simulink model "closed_circuited_cooling_tower_V2011"  (Simulink 7.0)
settings: Solver=ode45  StartTime=3600*24*250  StopTime=3600*24*260  RelTol=1e-3
libraries: carnot x8
settings Model: Creator=Mario  LastModifiedBy=Sandra  SimulationMode=accelerator

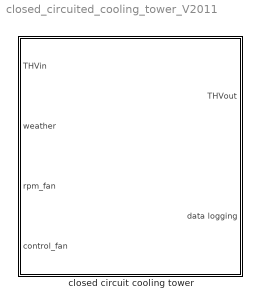
== system closed_circuited_cooling_tower_V2011 ==
  closed circuit cooling tower : Subsystem  AncestorBlock=carnot/misc/THV_template
      mask Type: Closed Circuit Cooling Tower
      mask Description:
      | performance data
      | wet-bulb temperature - 15°C ... 24°C
      | rpm fan - 248 1/min (30%) ... 824 1/min (100%)
      | fluid temperature - 26°C ... 44°C
      | fluid flow rate - 1,07 l/s ... 3,03 l/s
      | water/glykol - 0 % ... 100%
      | 
      | data logging:
      | wet-bulb temperature....[°C]   (ambient air)
      | rpm fan.........................[%]
      | v_dot fan......................[m³/s]
      | rpm fan.........................[1/min]
      | rel_hum.........................[%]     (ambient air)
      | t_air..............................[°C]    (ambient air)
      | energy ct......................[kJ]    (fan motor + recirculating spray pump)
      | power ct.......................[kW]    (fan motor + recirculating spray pump)
      | water consumption.......[kg]
      | Tnodes.........................[°C]    (inactivity modul)
      | THVout
      mask Display:
      | plot(-20,5,140,80,[20 90 90 20 20],[20 20 70 70 20])
      | plot([30 35],[62 65],[40 35],[62 65],[35 35],[62 65],[80 80],[62 65],[75 80],[62 65],[85 80],[62 65],[57 57],[62 65],[52 57],[62 65],[62 57],[62 65])
      | plot([15 20],[22 22],[15 80],[65 65],[15 15],[22 65],[20 90],[24 24])
      | plot([25 100],[58 58],[25 100],[44 44],[60 25],[51 58],[60 25],[51 44])
      | plot([87 93],[36 36],[87 93],[28 28],[87 82],[36 34],[93 98],[36 34],[87 82],[28 30],[93 98],[28 30],[82 82],[34 30],[98 98],[34 30],[82 95],[34 35],[82 95],[30 29])
      | plot([86 90],[32 32],[90 93],[32 33.5],[90 93],[32 30.5])

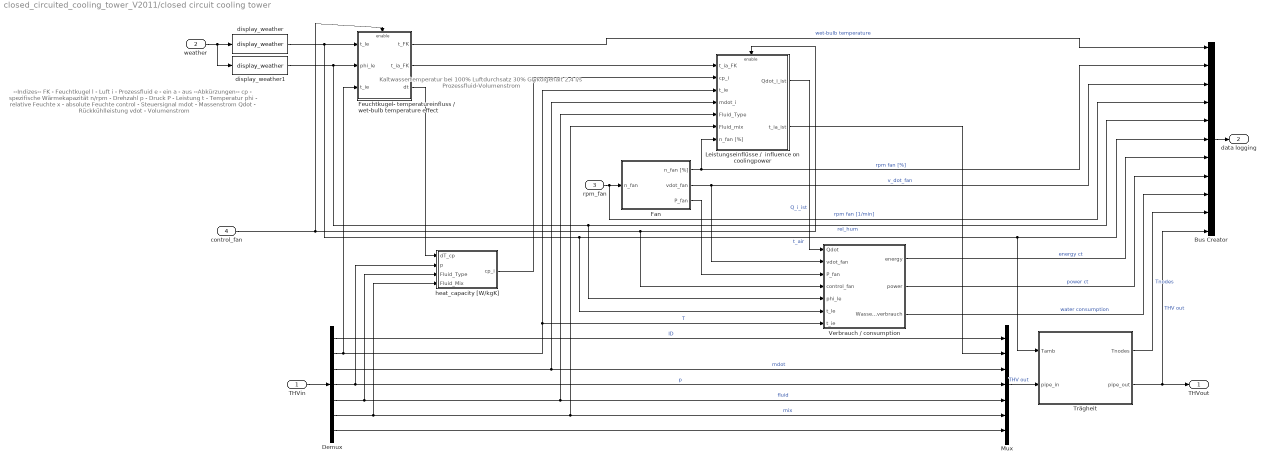
== system closed_circuited_cooling_tower_V2011/closed circuit cooling tower ==
  note: Kaltwassertemperatur bei
      | 100% Luftdurchsatz
      | 30% Glykolgehalt
      | 2,4 l/s Prozessfluid-Volumenstrom
  note: --Indizes--
      | FK - Feuchtkugel
      | l - Luft
      | i - Prozessfluid
      | e - ein
      | a - aus
      |
      |
      | --Abkürzungen--
      | cp - spezifische Wärmekapazität
      | n/rpm - Drehzahl
      | p - Druck
      | P - Leistung
      | t - Temperatur
      | phi - relative Feuchte
      | x - absolute Feuchte
      | control - Steuersignal
      | mdot - Massenstrom
      | Qdot - Rückkühlleistung
      | vdot - Volumenstrom
  THVin : Inport  OutDataType=sfix(16)  OutScaling=2^0
  weather : Inport  Port=2  OutDataType=sfix(16)  OutScaling=2^0
  rpm_fan : Inport  Port=3  OutDataType=sfix(16)  OutScaling=2^0
  control_fan : Inport  Port=4  OutDataType=sfix(16)  OutScaling=2^0
  Bus Creator : BusCreator  Inputs=11
  Demux : Demux  Outputs=[1 1 1 1 1 1 14]
  Fan : Subsystem  AncestorBlock=carnot/misc/THV_template
  Feuchtkugel- temperatureinfluss / wet-bulb temperature effect : Subsystem  AncestorBlock=carnot/misc/THV_template
  Leistungseinflüsse /  influence on coolingpower : Subsystem  AncestorBlock=carnot/misc/THV_template
  Mux : Mux  Inputs=7
  Trägheit : Subsystem  AncestorBlock=carnot/storage/storage_multiport_2  mask(storage with heat exchangers){diameter=0.1, vol=0.04, pos=standing cylinder, heatloss=7, hlossbot=7, axialcond=1.1, tinitial=21}
      mask prompts: diameter "diameter [m]"; vol "volume [m³]"; pos "position"; heatloss "heat loss coefficient wall [W/(m²*K)]"; hlossbot "heat loss coefficient bottom [W/(m²*K)]"; axialcond "effective axial conductivity in [W/(m*K)]"; tinitial "initial temperature [degree centigrade]"
      mask help:
      | Storage is a standing cylinder. It can be divided in several nodes.
      | Outputs can be refined up to nodes temperature sensors.
      | (See mask of storage in subsystem by <look under mask - command> for details of numerical properties).
      |
      | Axial conductivity includes the fluid and wall conductivity.
      | Heat losses are calculated also for top and bottom surfaces.
      mask Help: eval('man(''storage_multiport'')')
      mask StyleString: edit,edit,popup(lying cylinder|standing cylinder),edit,edit,edit,edit
      mask Display: plot(0,0,100,100,[36,36,40,50,54,54,50,40,36],[90,50,45,45,50,90,93,93,90],[36,51,40,51,36],[74,74,79,85,85],[36,51,44,51,36],[54,54,56,58,58])
  Verbrauch / consumption : Subsystem  AncestorBlock=carnot/misc/THV_template
  display_weather : carnot/outputs/display_weather  SystemSampleTime=-1  pos=off  rad=off  ta=on  ts=off  pre=off  rh=off  ci=off  p=off  ws=off  wd=off  col=off
  display_weather1 : carnot/outputs/display_weather  SystemSampleTime=-1  pos=off  rad=off  ta=off  ts=off  pre=off  rh=on  ci=off  p=off  ws=off  wd=off  col=off
  heat_capacity [W/kgK] : Subsystem  AncestorBlock=carnot/materials/heat_capacity
      mask Type: heat capacity
      mask Description:
      | Calculates the  heat_capacity of fluids [J/(kg*K)].
      | Calls calls the function "hcap" in the CARNOT library "carlib".
      | Definition of the fluid types
      | fluid-ID  material           remarks on fluid mix
      | 1           water              vapourcontent in the 2-phase region
      | 2           air                   is (kg water) / (kg air)
      | 3           cotton oil
      | 4           silicone oil
      | 5           water-glycol    gives the volume partition [0..1] of glycol
      mask Help: eval('htmlhelp (''chap_4_2h.htm#heat_capacity'')')
  THVout : Outport  OutDataType=sfix(16)  OutScaling=2^0  InitialOutput=0
  data logging : Outport  Port=2  OutDataType=sfix(16)  OutScaling=2^0  InitialOutput=0
  wires:
  THVin/1 -> Demux/1
  Demux/3 -> Leistungseinflüsse /  influence on coolingpower/4(mdot_i), Mux/3  "mdot"
  Demux/7 -> Mux/7
  Demux/5 -> heat_capacity [W/kgK]/3(Fluid_Type), Mux/5, Leistungseinflüsse /  influence on coolingpower/5(Fluid_Type)  "fluid"
  Mux/1 -> Trägheit/2(pipe_in)  "THV out"
  Demux/4 -> heat_capacity [W/kgK]/2(p), Mux/4  "p"
  rpm_fan/1 -> Fan/1(n_fan), Bus Creator/4  "rpm fan [1/min]"
  Feuchtkugel- temperatureinfluss / wet-bulb temperature effect/3(dt) -> heat_capacity [W/kgK]/1(dT_cp)
  Feuchtkugel- temperatureinfluss / wet-bulb temperature effect/2(t_ia_FK) -> Leistungseinflüsse /  influence on coolingpower/1(t_ia_FK)
  Demux/2 -> Feuchtkugel- temperatureinfluss / wet-bulb temperature effect/3(t_ie), Leistungseinflüsse /  influence on coolingpower/3(t_ie), Verbrauch / consumption/7(t_ie)  "T"
  Leistungseinflüsse /  influence on coolingpower/2(t_ia_ist) -> Mux/2
  heat_capacity [W/kgK]/1(cp_i) -> Leistungseinflüsse /  influence on coolingpower/2(cp_i)
  Fan/2(vdot_fan) -> Verbrauch / consumption/2(vdot_fan), Bus Creator/3  "v_dot_fan"
  Verbrauch / consumption/2(power) -> Bus Creator/8  "power ct"
  Fan/3(P_fan) -> Verbrauch / consumption/3(P_fan)
  control_fan/1 -> Verbrauch / consumption/4(control_fan), Leistungseinflüsse /  influence on coolingpower/Enable, Feuchtkugel- temperatureinfluss / wet-bulb temperature effect/Enable
  Demux/1 -> Mux/1  "ID"
  Feuchtkugel- temperatureinfluss / wet-bulb temperature effect/1(t_FK) -> Bus Creator/1  "wet-bulb temperature"
  Leistungseinflüsse /  influence on coolingpower/1(Qdot_i_ist) -> Verbrauch / consumption/1(Qdot)  "Q_i_ist"
  Fan/1(n_fan [%]) -> Leistungseinflüsse /  influence on coolingpower/7(n_fan [%]), Bus Creator/2  "rpm fan [%]"
  display_weather1/1 -> Feuchtkugel- temperatureinfluss / wet-bulb temperature effect/2(phi_le), Verbrauch / consumption/5(phi_le), Bus Creator/5  "rel_hum"
  display_weather/1 -> Feuchtkugel- temperatureinfluss / wet-bulb temperature effect/1(t_le), Verbrauch / consumption/6(t_le), Trägheit/1(Tamb), Bus Creator/6  "t_air"
  Verbrauch / consumption/3(Wasserverbrauch) -> Bus Creator/9  "water consumption"
  Trägheit/1(Tnodes) -> Bus Creator/10  "Tnodes"
  Trägheit/2(pipe_out) -> THVout/1, Bus Creator/11  "THV out"
  Demux/6 -> heat_capacity [W/kgK]/4(Fluid_Mix), Leistungseinflüsse /  influence on coolingpower/6(Fluid_mix), Mux/6  "mix"
  weather/1 -> display_weather/1, display_weather1/1
  Bus Creator/1 -> data logging/1
  Verbrauch / consumption/1(energy) -> Bus Creator/7  "energy ct"

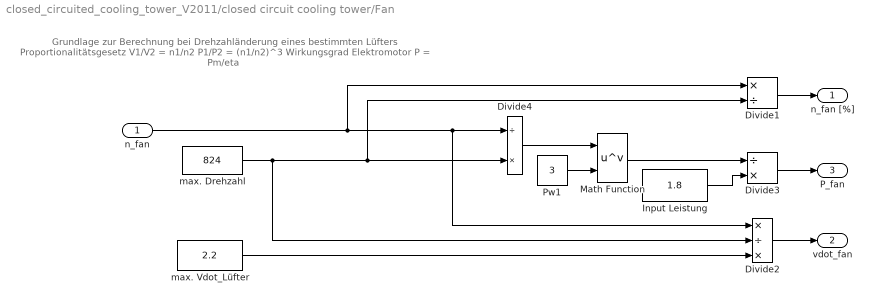
== system closed_circuited_cooling_tower_V2011/closed circuit cooling tower/Fan ==
  note: Grundlage zur Berechnung
      | bei Drehzahländerung eines bestimmten Lüfters
      |
      | Proportionalitätsgesetz
      | V1/V2 = n1/n2
      | P1/P2 = (n1/n2)^3
      |
      | Wirkungsgrad Elektromotor
      | P = Pm/eta
  n_fan : Inport  OutDataType=sfix(16)  OutScaling=2^0
  Divide1 : Product  Inputs=*/  OutDataType=sfix(16)  OutScaling=2^-10
  Divide2 : Product  Inputs=*/*  OutDataType=sfix(16)  OutScaling=2^-10
  Divide3 : Product  Inputs=/*  OutDataType=sfix(16)  OutScaling=2^-10
  Divide4 : Product  Inputs=/*  OutDataType=sfix(16)  OutScaling=2^-10
  Input Leistung : Constant  Value=1.8  OutDataType=sfix(16)  OutScaling=2^0
  Math Function : Math  Operator=pow  OutDataType=sfix(16)  OutScaling=2^0  SaturateOnIntegerOverflow=on
  Pw1 : Constant  Value=3  OutDataType=sfix(16)  OutScaling=2^0
  max. Drehzahl : Constant  Value=824  OutDataType=sfix(16)  OutScaling=2^0
  max. Vdot_Lüfter : Constant  Value=2.2  OutDataType=sfix(16)  OutScaling=2^0
  n_fan [%] : Outport  OutDataType=sfix(16)  OutScaling=2^0  InitialOutput=0
  vdot_fan : Outport  Port=2  OutDataType=sfix(16)  OutScaling=2^0  InitialOutput=0
  P_fan : Outport  Port=3  OutDataType=sfix(16)  OutScaling=2^0  InitialOutput=0
  wires:
  n_fan/1 -> Divide2/1, Divide4/1, Divide1/1
  max. Drehzahl/1 -> Divide2/2, Divide1/2, Divide4/2
  Divide1/1 -> n_fan [%]/1
  Input Leistung/1 -> Divide3/2
  max. Vdot_Lüfter/1 -> Divide2/3
  Divide2/1 -> vdot_fan/1
  Divide3/1 -> P_fan/1
  Divide4/1 -> Math Function/1
  Math Function/1 -> Divide3/1
  Pw1/1 -> Math Function/2

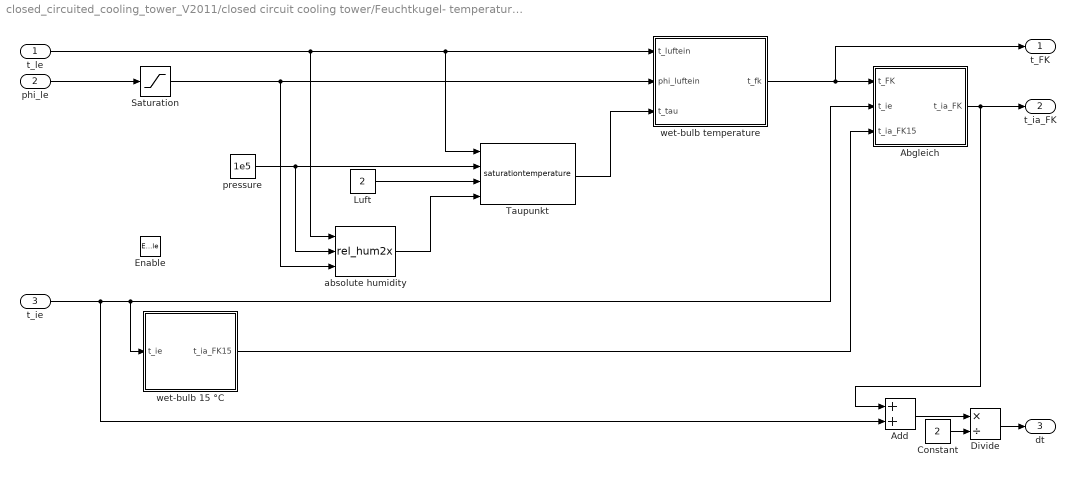
== system closed_circuited_cooling_tower_V2011/closed circuit cooling tower/Feuchtkugel- temperatureinfluss / wet-bulb temperature effect ==
  t_le : Inport  OutDataType=sfix(16)  OutScaling=2^0
  phi_le : Inport  Port=2  OutDataType=sfix(16)  OutScaling=2^0
  t_ie : Inport  Port=3  OutDataType=sfix(16)  OutScaling=2^0
  Enable : EnablePort
  "Abgleich " : Subsystem  AncestorBlock=carnot/misc/THV_template
  Add : Sum  OutDataType=sfix(16)  OutScaling=2^-10
  Constant : Constant  Value=2  OutDataType=sfix(16)  OutScaling=2^0
  Divide : Product  Inputs=*/  OutDataType=sfix(16)  OutScaling=2^-10
  Luft : Constant  Value=2  OutDataType=sfix(16)  OutScaling=2^0
  Saturation : Saturate  UpperLimit=99.0  LowerLimit=0  OutDataType=sfix(16)  OutScaling=2^0
  Taupunkt : carnot/materials/saturationtemperature  SystemSampleTime=-1
  absolute humidity : carnot/basics/rel_hum2x  SystemSampleTime=-1
  pressure : Constant  Value=1e5  OutDataType=sfix(16)  OutScaling=2^0
  wet-bulb 15 °C : Subsystem  AncestorBlock=carnot/misc/THV_template
  wet-bulb temperature : Stateflow chart
  t_FK : Outport  OutDataType=sfix(16)  OutScaling=2^0  InitialOutput=0
  t_ia_FK : Outport  Port=2  OutDataType=sfix(16)  OutScaling=2^0  InitialOutput=0
  dt : Outport  Port=3  OutDataType=sfix(16)  OutScaling=2^0  InitialOutput=0
  wires:
  wet-bulb 15 °C/1(t_ia_FK15) -> "Abgleich "/3(t_ia_FK15)
  wet-bulb temperature/1(t_fk) -> "Abgleich "/1(t_FK), t_FK/1
  t_ie/1 -> Add/2, wet-bulb 15 °C/1(t_ie), "Abgleich "/2(t_ie)
  phi_le/1 -> Saturation/1
  t_le/1 -> Taupunkt/1, wet-bulb temperature/1(t_luftein), absolute humidity/1
  "Abgleich "/1(t_ia_FK) -> Add/1, t_ia_FK/1
  Add/1 -> Divide/1
  Constant/1 -> Divide/2
  Divide/1 -> dt/1
  Saturation/1 -> absolute humidity/3, wet-bulb temperature/2(phi_luftein)
  absolute humidity/1 -> Taupunkt/4
  Luft/1 -> Taupunkt/3
  pressure/1 -> Taupunkt/2, absolute humidity/2
  Taupunkt/1 -> wet-bulb temperature/3(t_tau)

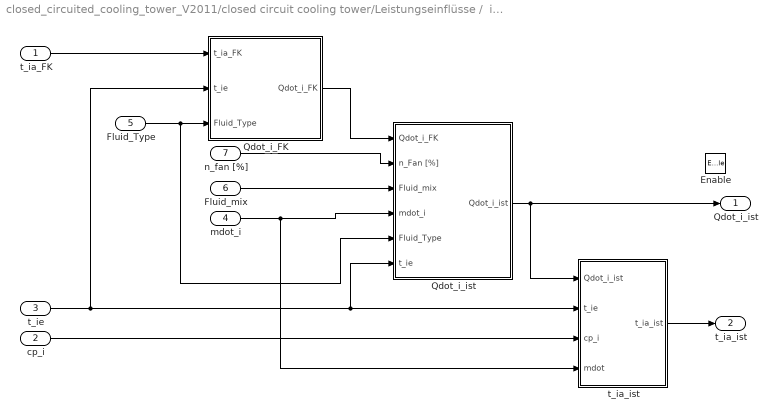
== system closed_circuited_cooling_tower_V2011/closed circuit cooling tower/Leistungseinflüsse /  influence on coolingpower ==
  t_ia_FK : Inport  OutDataType=sfix(16)  OutScaling=2^0
  cp_i : Inport  Port=2  OutDataType=sfix(16)  OutScaling=2^0
  t_ie : Inport  Port=3  OutDataType=sfix(16)  OutScaling=2^0
  mdot_i : Inport  Port=4  OutDataType=sfix(16)  OutScaling=2^0
  Fluid_Type : Inport  Port=5  OutDataType=sfix(16)  OutScaling=2^0
  Fluid_mix : Inport  Port=6  OutDataType=sfix(16)  OutScaling=2^0
  n_fan [%] : Inport  Port=7  OutDataType=sfix(16)  OutScaling=2^0
  Enable : EnablePort
  Qdot_i_FK : Subsystem  AncestorBlock=carnot/misc/THV_template
  "Qdot_i_ist " : Subsystem  AncestorBlock=carnot/misc/THV_template
  "t_ia_ist " : Subsystem  AncestorBlock=carnot/misc/THV_template
  Qdot_i_ist : Outport  OutDataType=sfix(16)  OutScaling=2^0  InitialOutput=0
  t_ia_ist : Outport  Port=2  OutDataType=sfix(16)  OutScaling=2^0  InitialOutput=0
  wires:
  "Qdot_i_ist "/1(Qdot_i_ist) -> Qdot_i_ist/1, "t_ia_ist "/1(Qdot_i_ist)
  Qdot_i_FK/1(Qdot_i_FK) -> "Qdot_i_ist "/1(Qdot_i_FK)
  t_ie/1 -> Qdot_i_FK/2(t_ie), "t_ia_ist "/2(t_ie), "Qdot_i_ist "/6(t_ie)
  t_ia_FK/1 -> Qdot_i_FK/1(t_ia_FK)
  n_fan [%]/1 -> "Qdot_i_ist "/2(n_Fan [%])
  "t_ia_ist "/1(t_ia_ist) -> t_ia_ist/1
  cp_i/1 -> "t_ia_ist "/3(cp_i)
  Fluid_Type/1 -> Qdot_i_FK/3(Fluid_Type), "Qdot_i_ist "/5(Fluid_Type)
  mdot_i/1 -> "Qdot_i_ist "/4(mdot_i), "t_ia_ist "/4(mdot)
  Fluid_mix/1 -> "Qdot_i_ist "/3(Fluid_mix)

== system closed_circuited_cooling_tower_V2011/closed circuit cooling tower/Trägheit ==
  Tamb : Inport  OutDataType=sfix(16)  OutScaling=2^0
  pipe_in : Inport  Port=2  OutDataType=sfix(16)  OutScaling=2^0
  Terminator : Terminator
  multiport storage : Subsystem  mask(internal mask of storage for numerical values){nodes=10, sensors=10, nport=1, d=[diameter vol], u=[heatloss hlossbot], axialcond=axialcond, tinitial=tinitial, pos=pos}
      mask prompts: nodes "number of nodes"; sensors "number of temperature sensors (first is at bottom)"; nport "number of ports"; d "geometry (DO NOT CHANGE HERE)"; u "heat losses (DO NOT CHANGE HERE)"; axialcond "effecive axial conductivity W/(m*K) (DO NOT CHANGE HERE)"; tinitial "initial temperature in °C (DO NOT CHANGE HERE)"; pos "position (DO NOT CHANGE HERE)"
      mask help: Model is one dimesional with <nodes> horizontal slices. Output sensor-temperatures are in equal distances over the storage (first output is lowest node).
      mask init:
      | nodes = max(nodes, 1);
      | sensors = max(sensors, 1);
      | d(1) = max(d(1), 0.001);
      | d(2) = max(d(2), 0.001);
      | pos = pos-1;
      mask Help:
      | The flow is calculated by the upwind scheme heat conduction between nodes by central diffenences (Patankar 1980).
      | Heat exchanger does not have any capacity for the fluid. Heat transfer to storage is calculated per stroage node by an energy balance. Heat transfer coefficient for heat exchanger is calculated from Nu = 0.5*(Gr*Pr)^0.25.
      | Can be charged and discharged by ports (straight incomming pipe, heat exchanger). For the moment You have to add the inports and outports yourself in  the subsystem when changing the number of ports. Be sure to keep the size of the demux after the s-funtion as [sensors 2  2  2] (repeat 2 as many ports as You have).
      mask StyleString: edit,edit,popup(1|2|3|4|5|6|7|8|9|10),edit,edit,edit,edit,edit
  pipe connection to store1 : Subsystem  AncestorBlock=carnot/storage/ports for your storage construction/pipe connection to store  mask(pipe connection to storage){hin=0, hout=1}
      mask prompts: hin "relative height of inlet"; hout "relative height of outlet"
      mask help:
      | The block transforms the incoming THV vector to a vector which the storage interprets as a flow into the storage fluid.
      | Give inlet- and outlet-height as a relative position from 0 (= bottom) to 1 (= top).
      mask init:
      | hin = min(1, max(0, hin));
      | hout = min(1, max(0, hout));
      mask Help: eval('man(''pipe_connection_to_store'')')
  Tnodes : Outport  OutDataType=sfix(16)  OutScaling=2^0  InitialOutput=0
  pipe_out : Outport  Port=2  OutDataType=sfix(16)  OutScaling=2^0  InitialOutput=0
  wires:
  multiport storage/2(Energy) -> Terminator/1
  pipe_in/1 -> pipe connection to store1/2(THVin)
  pipe connection to store1/2(THVout) -> pipe_out/1
  Tamb/1 -> multiport storage/1(Tamb)
  multiport storage/1(Tnodes) -> Tnodes/1
  multiport storage/3("[T p]1") -> pipe connection to store1/1(from store)
  pipe connection to store1/1(to store) -> multiport storage/2(port1)

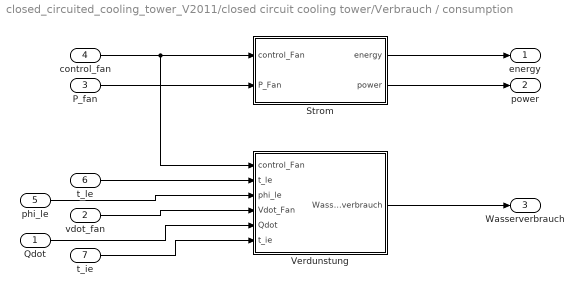
== system closed_circuited_cooling_tower_V2011/closed circuit cooling tower/Verbrauch / consumption ==
  Qdot : Inport  OutDataType=sfix(16)  OutScaling=2^0
  vdot_fan : Inport  Port=2  OutDataType=sfix(16)  OutScaling=2^0
  P_fan : Inport  Port=3  OutDataType=sfix(16)  OutScaling=2^0
  control_fan : Inport  Port=4  OutDataType=sfix(16)  OutScaling=2^0
  phi_le : Inport  Port=5  OutDataType=sfix(16)  OutScaling=2^0
  t_le : Inport  Port=6  OutDataType=sfix(16)  OutScaling=2^0
  t_ie : Inport  Port=7  OutDataType=sfix(16)  OutScaling=2^0
  Strom : Subsystem  AncestorBlock=carnot/misc/THV_template
  Verdunstung : Subsystem  AncestorBlock=carnot/misc/THV_template
  energy : Outport  OutDataType=sfix(16)  OutScaling=2^0  InitialOutput=0
  power : Outport  Port=2  OutDataType=sfix(16)  OutScaling=2^0  InitialOutput=0
  Wasserverbrauch : Outport  Port=3  OutDataType=sfix(16)  OutScaling=2^0  InitialOutput=0
  wires:
  control_fan/1 -> Strom/1(control_Fan), Verdunstung/1(control_Fan)
  P_fan/1 -> Strom/2(P_Fan)
  Strom/2(power) -> power/1
  t_le/1 -> Verdunstung/2(t_le)
  Verdunstung/1(Wasserverbrauch) -> Wasserverbrauch/1
  phi_le/1 -> Verdunstung/3(phi_le)
  vdot_fan/1 -> Verdunstung/4(Vdot_Fan)
  Qdot/1 -> Verdunstung/5(Qdot)
  t_ie/1 -> Verdunstung/6(t_ie)
  Strom/1(energy) -> energy/1

== system closed_circuited_cooling_tower_V2011/closed circuit cooling tower/heat_capacity [W/kgK] ==
  dT_cp : Inport  OutDataType=sfix(16)  OutScaling=2^0
  p : Inport  Port=2  OutDataType=sfix(16)  OutScaling=2^0
  Fluid_Type : Inport  Port=3  OutDataType=sfix(16)  OutScaling=2^0
  Fluid_Mix : Inport  Port=4  OutDataType=sfix(16)  OutScaling=2^0
  S-Function : S-Function  FunctionName=capfluid
  cp_i : Outport  OutDataType=sfix(16)  OutScaling=2^0  InitialOutput=0
  wires:
  S-Function/1 -> cp_i/1
  Fluid_Type/1 -> S-Function/1
  Fluid_Mix/1 -> S-Function/2
  dT_cp/1 -> S-Function/3
  p/1 -> S-Function/4

== system closed_circuited_cooling_tower_V2011/closed circuit cooling tower/Feuchtkugel- temperatureinfluss / wet-bulb temperature effect/Abgleich  ==
  note: Durch den Abgleich der vorliegenden Datensätze
      | wierd die Annahme getroffen
      | das bei einer reduzierung der Feuchtkugeltemp um 1K
      |  sich die Kaltwassertemp um 0.27K sinkt.
      |
      | y = ((t_FK-15)*0.27)+t_ia_100
      |
      | Ab eine Eintritstemperatur von 41 °C wierd mit
      | dem Faktor 0,25 K gerechnet.
      |
      | y = ((t_FK-15)*0.25)+t_ia_100
  t_FK : Inport  OutDataType=sfix(16)  OutScaling=2^0
  t_ie : Inport  Port=2  OutDataType=sfix(16)  OutScaling=2^0
  t_ia_FK15 : Inport  Port=3  OutDataType=sfix(16)  OutScaling=2^0
  Embedded MATLAB Function : Stateflow chart
  t_ia_FK : Outport  OutDataType=sfix(16)  OutScaling=2^0  InitialOutput=0
  wires:
  Embedded MATLAB Function/1(y) -> t_ia_FK/1
  t_FK/1 -> Embedded MATLAB Function/1(t_fk)
  t_ia_FK15/1 -> Embedded MATLAB Function/2(t_ia_fk15)
  t_ie/1 -> Embedded MATLAB Function/3(t_ie)

== system closed_circuited_cooling_tower_V2011/closed circuit cooling tower/Feuchtkugel- temperatureinfluss / wet-bulb temperature effect/wet-bulb 15 °C ==
  t_ie : Inport  OutDataType=sfix(16)  OutScaling=2^0
  Lookup Table : Lookup  InputValues=[26 28 30 32 34 36 38 40 42 44 79.2]  Table=[22.6 23.9 25.2 26.4 27.7 28.9 30.1 31.2 32.4 33.5 49.25]  OutDataType=sfix(16)  OutScaling=2^0
  t_ia_FK15 : Outport  OutDataType=sfix(16)  OutScaling=2^0  InitialOutput=0
  wires:
  t_ie/1 -> Lookup Table/1
  Lookup Table/1 -> t_ia_FK15/1

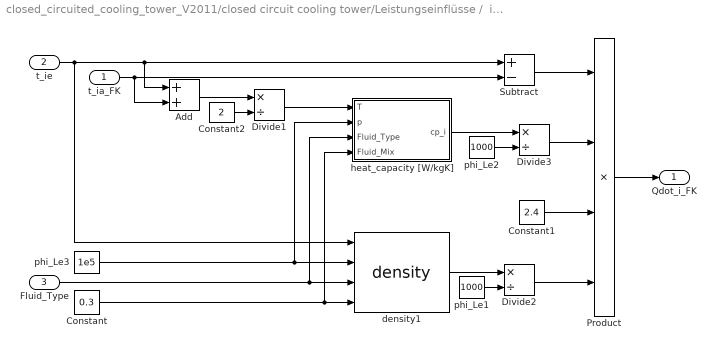
== system closed_circuited_cooling_tower_V2011/closed circuit cooling tower/Leistungseinflüsse /  influence on coolingpower/Qdot_i_FK ==
  t_ia_FK : Inport  OutDataType=sfix(16)  OutScaling=2^0
  t_ie : Inport  Port=2  OutDataType=sfix(16)  OutScaling=2^0
  Fluid_Type : Inport  Port=3  OutDataType=sfix(16)  OutScaling=2^0
  Add : Sum  OutDataType=sfix(16)  OutScaling=2^-10
  Constant : Constant  Value=0.3  OutDataType=sfix(16)  OutScaling=2^0
  Constant1 : Constant  Value=2.4  OutDataType=sfix(16)  OutScaling=2^0
  Constant2 : Constant  Value=2  OutDataType=sfix(16)  OutScaling=2^0
  Divide1 : Product  Inputs=*/  OutDataType=sfix(16)  OutScaling=2^-10
  Divide2 : Product  Inputs=*/  OutDataType=sfix(16)  OutScaling=2^-10
  Divide3 : Product  Inputs=*/  OutDataType=sfix(16)  OutScaling=2^-10
  Product : Product  Inputs=4  OutDataType=sfix(16)  OutScaling=2^0  RndMeth=Zero
  Subtract : Sum  Inputs=+-  OutDataType=sfix(16)  OutScaling=2^-10
  density1 : carnot/materials/density  SystemSampleTime=-1
  heat_capacity [W/kgK] : Subsystem  AncestorBlock=carnot/materials/heat_capacity
      mask Type: heat capacity
      mask Description:
      | Calculates the  heat_capacity of fluids [J/(kg*K)].
      | Calls calls the function "hcap" in the CARNOT library "carlib".
      | Definition of the fluid types
      | fluid-ID  material           remarks on fluid mix
      | 1           water              vapourcontent in the 2-phase region
      | 2           air                   is (kg water) / (kg air)
      | 3           cotton oil
      | 4           silicone oil
      | 5           water-glycol    gives the volume partition [0..1] of glycol
      mask Help: eval('htmlhelp (''chap_4_2h.htm#heat_capacity'')')
  phi_Le1 : Constant  Value=1000  OutDataType=sfix(16)  OutScaling=2^0
  phi_Le2 : Constant  Value=1000  OutDataType=sfix(16)  OutScaling=2^0
  phi_Le3 : Constant  Value=1e5  OutDataType=sfix(16)  OutScaling=2^0
  Qdot_i_FK : Outport  OutDataType=sfix(16)  OutScaling=2^0  InitialOutput=0
  wires:
  t_ia_FK/1 -> Subtract/2, Add/2
  Product/1 -> Qdot_i_FK/1
  Subtract/1 -> Product/1
  t_ie/1 -> density1/1, Subtract/1, Add/1
  Constant/1 -> density1/4, heat_capacity [W/kgK]/4(Fluid_Mix)
  density1/1 -> Divide2/1
  phi_Le3/1 -> density1/2, heat_capacity [W/kgK]/2(p)
  Fluid_Type/1 -> density1/3, heat_capacity [W/kgK]/3(Fluid_Type)
  phi_Le1/1 -> Divide2/2
  Divide2/1 -> Product/4
  Constant1/1 -> Product/3
  heat_capacity [W/kgK]/1(cp_i) -> Divide3/1
  Constant2/1 -> Divide1/2
  Divide1/1 -> heat_capacity [W/kgK]/1(T)
  Add/1 -> Divide1/1
  phi_Le2/1 -> Divide3/2
  Divide3/1 -> Product/2

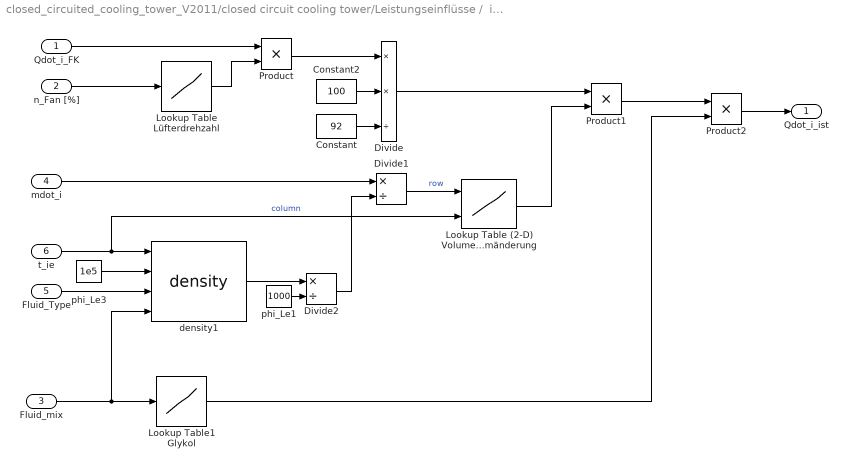
== system closed_circuited_cooling_tower_V2011/closed circuit cooling tower/Leistungseinflüsse /  influence on coolingpower/Qdot_i_ist  ==
  Qdot_i_FK : Inport  OutDataType=sfix(16)  OutScaling=2^0
  n_Fan [%] : Inport  Port=2  OutDataType=sfix(16)  OutScaling=2^0
  Fluid_mix : Inport  Port=3  OutDataType=sfix(16)  OutScaling=2^0
  mdot_i : Inport  Port=4  OutDataType=sfix(16)  OutScaling=2^0
  Fluid_Type : Inport  Port=5  OutDataType=sfix(16)  OutScaling=2^0
  t_ie : Inport  Port=6  OutDataType=sfix(16)  OutScaling=2^0
  Constant : Constant  Value=92  OutDataType=sfix(16)  OutScaling=2^0
  Constant2 : Constant  Value=100  OutDataType=sfix(16)  OutScaling=2^0
  Divide : Product  Inputs=**/  OutDataType=sfix(16)  OutScaling=2^-10
  Divide1 : Product  Inputs=*/  OutDataType=sfix(16)  OutScaling=2^-10
  Divide2 : Product  Inputs=*/  OutDataType=sfix(16)  OutScaling=2^-10
  Lookup Table (2-D) Volumenstromänderung : Lookup2D  RowIndex=[1.07 1.77 2.4 2.65 3.03]  ColumnIndex=[25 30 35 40 45 50 55 60 65]  Table=[0.7248 0.7054 0.6860 0.6666 0.6472 0.6278 0.6084 0.5890 0.5696; 0.9493 0.9294 0.9096 0.8897 0.8698 0.8500 0.8301 0.8103 0.7904; 1 1 1 1 1 1 1 1 1; 1.1191 1.1295 1.0956 1.0674 1.0450 1.0284 1.0175 1.0123 1.0129; 1.2370 1.1910 1.1526 1.1219 1.0988 1.0833 1.0754 1.0752 1.0826]  OutDataType=sfix(16)  OutScaling=2^0
  Lookup Table Lüfterdrehzahl : Lookup  InputValues=[0 0.2 0.3 0.5 0.7 0.9 1]  Table=[0 0.37 0.482 0.625 0.786 0.928 1]  OutDataType=sfix(16)  OutScaling=2^0
  Lookup Table1 Glykol : Lookup  InputValues=[0 0.1 0.2 0.3 0.4 0.5 0.6 0.7 0.8 0.9 1]  Table=[1 0.98 0.95 0.92 0.875 0.83 0.78 0.73 0.68 0.63 0.57]  OutDataType=sfix(16)  OutScaling=2^0
  Product : Product  OutDataType=sfix(16)  OutScaling=2^0  RndMeth=Zero
  Product1 : Product  OutDataType=sfix(16)  OutScaling=2^0  RndMeth=Zero
  Product2 : Product  OutDataType=sfix(16)  OutScaling=2^0  RndMeth=Zero
  density1 : carnot/materials/density  SystemSampleTime=-1
  phi_Le1 : Constant  Value=1000  OutDataType=sfix(16)  OutScaling=2^0
  phi_Le3 : Constant  Value=1e5  OutDataType=sfix(16)  OutScaling=2^0
  Qdot_i_ist : Outport  OutDataType=sfix(16)  OutScaling=2^0  InitialOutput=0
  wires:
  n_Fan [%]/1 -> Lookup Table Lüfterdrehzahl/1
  Lookup Table Lüfterdrehzahl/1 -> Product/2
  Qdot_i_FK/1 -> Product/1
  Product/1 -> Divide/1
  Product1/1 -> Product2/1
  Lookup Table1 Glykol/1 -> Product2/2
  Fluid_mix/1 -> density1/4, Lookup Table1 Glykol/1
  Divide/1 -> Product1/1
  Constant/1 -> Divide/3
  mdot_i/1 -> Divide1/1
  Product2/1 -> Qdot_i_ist/1
  density1/1 -> Divide2/1
  phi_Le3/1 -> density1/2
  Fluid_Type/1 -> density1/3
  phi_Le1/1 -> Divide2/2
  Divide2/1 -> Divide1/2
  t_ie/1 -> density1/1, Lookup Table (2-D) Volumenstromänderung/2  "column"
  Divide1/1 -> Lookup Table (2-D) Volumenstromänderung/1  "row"
  Lookup Table (2-D) Volumenstromänderung/1 -> Product1/2
  Constant2/1 -> Divide/2

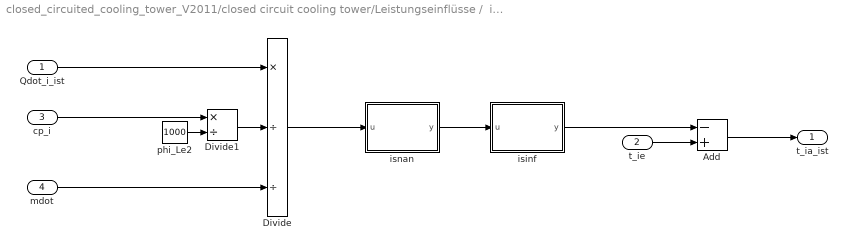
== system closed_circuited_cooling_tower_V2011/closed circuit cooling tower/Leistungseinflüsse /  influence on coolingpower/t_ia_ist  ==
  Qdot_i_ist : Inport  OutDataType=sfix(16)  OutScaling=2^0
  t_ie : Inport  Port=2  OutDataType=sfix(16)  OutScaling=2^0
  cp_i : Inport  Port=3  OutDataType=sfix(16)  OutScaling=2^0
  mdot : Inport  Port=4  OutDataType=sfix(16)  OutScaling=2^0
  Add : Sum  Inputs=-+  OutDataType=sfix(16)  OutScaling=2^-10
  Divide : Product  Inputs=*//  OutDataType=sfix(16)  OutScaling=2^-10
  Divide1 : Product  Inputs=*/  OutDataType=sfix(16)  OutScaling=2^-10
  isinf : Stateflow chart
  isnan : Stateflow chart
  phi_Le2 : Constant  Value=1000  OutDataType=sfix(16)  OutScaling=2^0
  t_ia_ist : Outport  OutDataType=sfix(16)  OutScaling=2^0  InitialOutput=0
  wires:
  Add/1 -> t_ia_ist/1
  Qdot_i_ist/1 -> Divide/1
  t_ie/1 -> Add/2
  Divide/1 -> isnan/1(u)
  cp_i/1 -> Divide1/1
  isnan/1(y) -> isinf/1(u)
  phi_Le2/1 -> Divide1/2
  Divide1/1 -> Divide/2
  mdot/1 -> Divide/3
  isinf/1(y) -> Add/1

== system closed_circuited_cooling_tower_V2011/closed circuit cooling tower/Trägheit/multiport storage ==
  Tamb : Inport  OutDataType=sfix(16)  OutScaling=2^0
  port1 : Inport  Port=2  OutDataType=sfix(16)  OutScaling=2^0
  S-Function : S-Function  FunctionName=store_hx  Parameters="d(1), d(2),  pos, u(1), u(2),  axialcond,  tinitial,  nodes, nport, sensors"
  Tnodes : Outport  OutDataType=sfix(16)  OutScaling=2^0  InitialOutput=0
  Energy : Outport  Port=2  OutDataType=sfix(16)  OutScaling=2^0  InitialOutput=0
  "[T p]1" : Outport  Port=3  OutDataType=sfix(16)  OutScaling=2^0  InitialOutput=0
  wires:
  S-Function/2 -> Energy/1
  S-Function/3 -> "[T p]1"/1
  S-Function/1 -> Tnodes/1
  port1/1 -> S-Function/2
  Tamb/1 -> S-Function/1

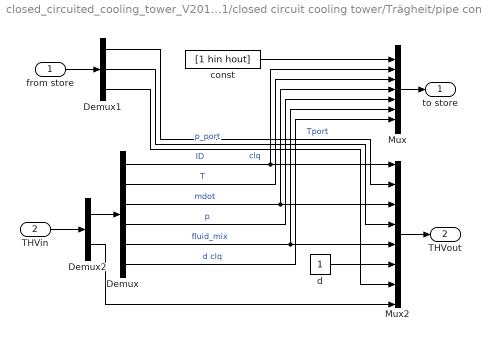
== system closed_circuited_cooling_tower_V2011/closed circuit cooling tower/Trägheit/pipe connection to store1 ==
  from store : Inport  OutDataType=sfix(16)  OutScaling=2^0
  THVin : Inport  Port=2  OutDataType=sfix(16)  OutScaling=2^0
  Demux : Demux  Outputs=[1 1 1 1 2 4]
  Demux1 : Demux  Outputs=[1 1 3]
  Demux2 : Demux  Outputs=[10 -1]
  Mux : Mux  Inputs=7
  Mux2 : Mux  Inputs=8
  const : Constant  Value=[1 hin hout]  OutDataType=sfix(16)  OutScaling=2^0
  d : Constant  OutDataType=sfix(16)  OutScaling=2^0
  to store : Outport  OutDataType=sfix(16)  OutScaling=2^0  InitialOutput=0
  THVout : Outport  Port=2  OutDataType=sfix(16)  OutScaling=2^0  InitialOutput=0
  wires:
  Demux/1 -> Mux/2, Mux2/1  "ID"
  from store/1 -> Demux1/1
  Demux2/1 -> Demux/1
  THVin/1 -> Demux2/1
  Demux/6 -> Mux/7  "d clq"
  Demux/5 -> Mux/6, Mux2/5  "fluid_mix"
  Demux/4 -> Mux/5  "p"
  Demux/3 -> Mux2/3, Mux/4  "mdot"
  Demux/2 -> Mux/3  "T"
  d/1 -> Mux2/6
  const/1 -> Mux/1
  Demux1/2 -> Mux2/4  "p_port"
  Demux1/1 -> Mux2/2  "Tport"
  Demux2/2 -> Mux2/8
  Demux1/3 -> Mux2/7  "clq"
  Mux/1 -> to store/1
  Mux2/1 -> THVout/1

== system closed_circuited_cooling_tower_V2011/closed circuit cooling tower/Verbrauch / consumption/Strom ==
  control_Fan : Inport  OutDataType=sfix(16)  OutScaling=2^0
  P_Fan : Inport  Port=2  OutDataType=sfix(16)  OutScaling=2^0
  Add : Sum  OutDataType=sfix(16)  OutScaling=2^-10
  Integrator1 : Integrator
  Product : Product  OutDataType=sfix(16)  OutScaling=2^0  RndMeth=Zero
  Product2 : Product  Inputs=*/  SaturateOnIntegerOverflow=on  RndMeth=Zero  InputSameDT=on
  Rieselwasserpumpe [kW] : Constant  Value=0.25  OutDataType=sfix(16)  OutScaling=2^0
  factor1 : Constant  Value=3600
  energy : Outport  OutDataType=sfix(16)  OutScaling=2^0  InitialOutput=0
  power : Outport  Port=2  OutDataType=sfix(16)  OutScaling=2^0  InitialOutput=0
  wires:
  Rieselwasserpumpe [kW]/1 -> Add/1
  Product/1 -> power/1, Integrator1/1
  control_Fan/1 -> Product/1
  Add/1 -> Product/2
  P_Fan/1 -> Add/2
  Integrator1/1 -> Product2/1
  factor1/1 -> Product2/2
  Product2/1 -> energy/1

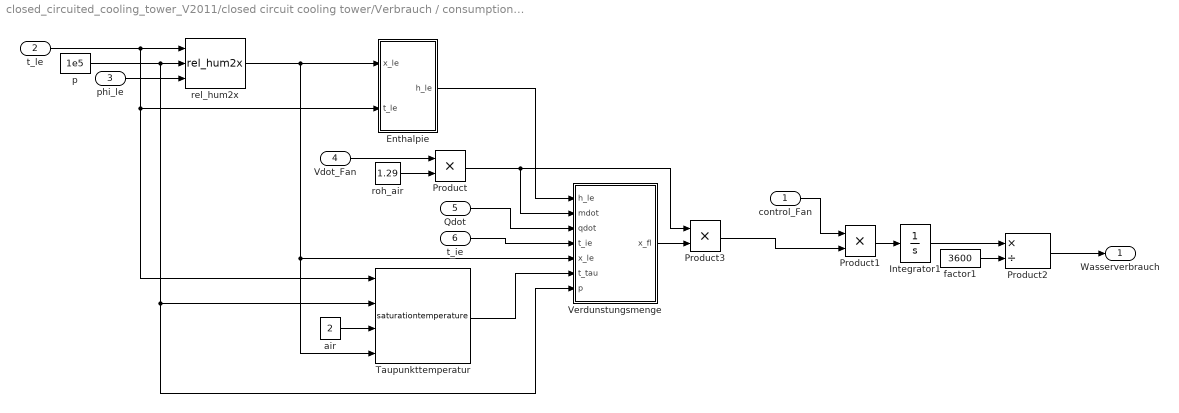
== system closed_circuited_cooling_tower_V2011/closed circuit cooling tower/Verbrauch / consumption/Verdunstung ==
  control_Fan : Inport  OutDataType=sfix(16)  OutScaling=2^0
  t_le : Inport  Port=2  OutDataType=sfix(16)  OutScaling=2^0
  phi_le : Inport  Port=3  OutDataType=sfix(16)  OutScaling=2^0
  Vdot_Fan : Inport  Port=4  OutDataType=sfix(16)  OutScaling=2^0
  Qdot : Inport  Port=5  OutDataType=sfix(16)  OutScaling=2^0
  t_ie : Inport  Port=6  OutDataType=sfix(16)  OutScaling=2^0
  "Enthalpie " : Subsystem  AncestorBlock=carnot/misc/THV_template
  Integrator1 : Integrator
  Product : Product  OutDataType=sfix(16)  OutScaling=2^0  RndMeth=Zero
  Product1 : Product  OutDataType=sfix(16)  OutScaling=2^0  RndMeth=Zero
  Product2 : Product  Inputs=*/  SaturateOnIntegerOverflow=on  RndMeth=Zero  InputSameDT=on
  Product3 : Product  OutDataType=sfix(16)  OutScaling=2^0  RndMeth=Zero
  Taupunkttemperatur : carnot/materials/saturationtemperature  SystemSampleTime=-1
  Verdunstungsmenge : Stateflow chart
  air : Constant  Value=2  OutDataType=sfix(16)  OutScaling=2^0
  factor1 : Constant  Value=3600
  p : Constant  Value=1e5  OutDataType=sfix(16)  OutScaling=2^0
  rel_hum2x : carnot/basics/rel_hum2x  SystemSampleTime=-1
  roh_air : Constant  Value=1.29  OutDataType=sfix(16)  OutScaling=2^0
  Wasserverbrauch : Outport  OutDataType=sfix(16)  OutScaling=2^0  InitialOutput=0
  wires:
  t_le/1 -> rel_hum2x/1, Taupunkttemperatur/1, "Enthalpie "/2(t_le)
  p/1 -> rel_hum2x/2, Taupunkttemperatur/2, Verdunstungsmenge/7(p)
  phi_le/1 -> rel_hum2x/3
  Vdot_Fan/1 -> Product/1
  roh_air/1 -> Product/2
  "Enthalpie "/1(h_le) -> Verdunstungsmenge/1(h_le)
  rel_hum2x/1 -> "Enthalpie "/1(x_le), Taupunkttemperatur/4, Verdunstungsmenge/5(x_le)
  Qdot/1 -> Verdunstungsmenge/3(qdot)
  Taupunkttemperatur/1 -> Verdunstungsmenge/6(t_tau)
  air/1 -> Taupunkttemperatur/3
  Integrator1/1 -> Product2/1
  factor1/1 -> Product2/2
  Product2/1 -> Wasserverbrauch/1
  Product1/1 -> Integrator1/1
  control_Fan/1 -> Product1/1
  Product3/1 -> Product1/2
  Product/1 -> Verdunstungsmenge/2(mdot), Product3/1
  t_ie/1 -> Verdunstungsmenge/4(t_ie)
  Verdunstungsmenge/1(x_fl) -> Product3/2

== system closed_circuited_cooling_tower_V2011/closed circuit cooling tower/Leistungseinflüsse /  influence on coolingpower/Qdot_i_FK/heat_capacity [W/kgK] ==
  T : Inport  OutDataType=sfix(16)  OutScaling=2^0
  p : Inport  Port=2  OutDataType=sfix(16)  OutScaling=2^0
  Fluid_Type : Inport  Port=3  OutDataType=sfix(16)  OutScaling=2^0
  Fluid_Mix : Inport  Port=4  OutDataType=sfix(16)  OutScaling=2^0
  S-Function : S-Function  FunctionName=capfluid
  cp_i : Outport  OutDataType=sfix(16)  OutScaling=2^0  InitialOutput=0
  wires:
  S-Function/1 -> cp_i/1
  Fluid_Type/1 -> S-Function/1
  Fluid_Mix/1 -> S-Function/2
  T/1 -> S-Function/3
  p/1 -> S-Function/4

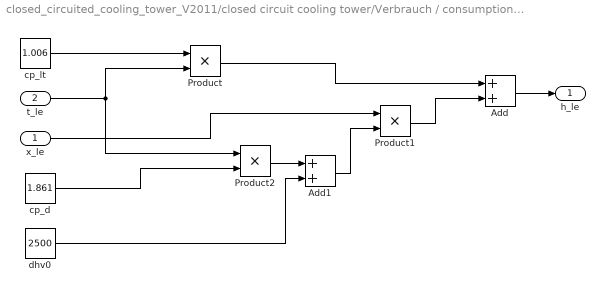
== system closed_circuited_cooling_tower_V2011/closed circuit cooling tower/Verbrauch / consumption/Verdunstung/Enthalpie  ==
  x_le : Inport  OutDataType=sfix(16)  OutScaling=2^0
  t_le : Inport  Port=2  OutDataType=sfix(16)  OutScaling=2^0
  Add : Sum  OutDataType=sfix(16)  OutScaling=2^-10
  Add1 : Sum  OutDataType=sfix(16)  OutScaling=2^-10
  Product : Product  OutDataType=sfix(16)  OutScaling=2^0  RndMeth=Zero
  Product1 : Product  OutDataType=sfix(16)  OutScaling=2^0  RndMeth=Zero
  Product2 : Product  OutDataType=sfix(16)  OutScaling=2^0  RndMeth=Zero
  cp_d : Constant  Value=1.861  OutDataType=sfix(16)  OutScaling=2^0
  cp_lt : Constant  Value=1.006  OutDataType=sfix(16)  OutScaling=2^0
  dhv0 : Constant  Value=2500  OutDataType=sfix(16)  OutScaling=2^0
  h_le : Outport  OutDataType=sfix(16)  OutScaling=2^0  InitialOutput=0
  wires:
  Add/1 -> h_le/1
  cp_lt/1 -> Product/1
  t_le/1 -> Product/2, Product2/1
  Product/1 -> Add/1
  Product1/1 -> Add/2
  x_le/1 -> Product1/1
  cp_d/1 -> Product2/2
  Add1/1 -> Product1/2
  Product2/1 -> Add1/1
  dhv0/1 -> Add1/2

== matlab function closed circuit cooling tower/Feuchtkugel- temperatureinfluss / wet-bulb temperature effect/Abgleich /Embedded MATLAB Function ==
  data: t_fk input inherited; y output inherited; t_ia_fk15 input inherited; t_ie input inherited
%Festlegung der Eingänge
function y = fcn(t_fk, t_ia_fk15, t_ie)

%Änderung des Faktors
if t_ie < 41
    
    y = ((t_fk-15)*0.27)+t_ia_fk15;
    
else
    
    y = ((t_fk-15)*0.25)+t_ia_fk15;
    
end

== matlab function closed circuit cooling tower/Feuchtkugel- temperatureinfluss / wet-bulb temperature effect/wet-bulb temperature ==
  data: t_luftein input inherited; t_fk output inherited; phi_luftein input inherited; t_tau input inherited
%Festlegung der Eingänge
function t_fk = fcn(t_luftein, phi_luftein, t_tau)

%Konstante/Variable
cp_luft = 1.006;        %[kJ/kgK]
cp_dampf = 1.861;       %[kJ/kgK]
cp_wasser = 4.19;       %[kJ/kgK]
dh_v0 = 2500;           %[kJ/kg]
phi_feuchtkugel = 100;  %[%]
p = 10^5;               %[Pa]
m = 1;
tmax = t_luftein;       %[°C]
tmin = t_tau;           %[°C]

% Absolute Feuchte-Berechnung Lufteintritt Bereich 0°C < t < 100°C [1]
ps_luftein = 611*exp((-1.91275)*10^(-4)+7.258*10^(-2)*t_luftein-2.939*10^(-4)*t_luftein^2+9.841*10^(-7)*t_luftein^3-1.92*10^(-9)*t_luftein^4);
x_luftein = (0.622*(phi_luftein/100)*ps_luftein)/(p-(phi_luftein/100)*ps_luftein);

% Enthalpieberechnung Lufteintritt
h_luftein = cp_luft*t_luftein+x_luftein*(cp_dampf*t_luftein+dh_v0);

% Feuchtkugeltemperaturberechnung, Halbierungsverfahren
t_feuchtkugel = (tmax+tmin)/2;

% Absolute Feuchteberechnung Feuchtkugel Bereich 0°C < t < 100°C [1]
ps_feuchtkugel = 611*exp((-1.91275)*10^(-4)+7.258*10^(-2)*t_feuchtkugel-2.939*10^(-4)*t_feuchtkugel^2+9.841*10^(-7)*t_feuchtkugel^3-1.92*10^(-9)*t_feuchtkugel^4);
x_feuchtkugel = (0.622*(phi_feuchtkugel/100)*ps_feuchtkugel)/(p-(phi_feuchtkugel/100)*ps_feuchtkugel);

% Enthalpieberechnung Feuchtkugel
h_feuchtkugel = cp_luft*t_feuchtkugel+x_feuchtkugel*(cp_dampf*t_feuchtkugel+dh_v0);

% Berechnung der Werte u1 und u2,; Formel aus VDI-Wärmeatlas
u1 = (h_luftein-h_feuchtkugel)/(x_luftein-x_feuchtkugel);
u2 = cp_wasser*t_feuchtkugel;

% Bewertung von u1 und u2 Beginn der Schleife
%            (u1-u2)<=0.001 ist die Feuchtkugeltemperatur gefunden
%            u1>u2 tmax = tFk
%            u1<u2 tmin = tFk
 while (u1-u2)>0.001 || (u1-u2)< 0 
    
    if u1>u2
        tmax = t_feuchtkugel;
        
    else 
        tmin = t_feuchtkugel;
        
    end
  
% Feuchtkugeltemperaturberechnung
t_feuchtkugel = (tmax+tmin)/2;

% Absolute Feuchteberechnung Feuchtkugel
ps_feuchtkugel = 611*exp((-1.91275)*10^(-4)+7.258*10^(-2)*t_feuchtkugel-2.939*10^(-4)*t_feuchtkugel^2+9.841*10^(-7)*t_feuchtkugel^3-1.92*10^(-9)*t_feuchtkugel^4);
x_feuchtkugel = (0.622*(phi_feuchtkugel/100)*ps_feuchtkugel)/(p-(phi_feuchtkugel/100)*ps_feuchtkugel);

% Enthalpieberechnung Feuchtkugel
h_feuchtkugel = cp_luft*t_feuchtkugel+x_feuchtkugel*(cp_dampf*t_feuchtkugel+dh_v0);

% Berechnung der Werte u1 und u2
u1 = (h_luftein-h_feuchtkugel)/(x_luftein-x_feuchtkugel);
u2 = cp_wasser*t_feuchtkugel;

% Schleifenzähler
m = m+1;
 
end

% Feuchtkugeltemperatur gefunden - Ausgabe
t_fk = t_feuchtkugel;

== matlab function closed circuit cooling tower/Leistungseinflüsse / influence on coolingpower/t_ia_ist /isinf ==
  data: u input inherited; y output inherited

function y = fcn(u)

%Verhindert die Fehlerausgabe bei Teilen mit dem Wert 0 
%Dieser Zustand tritt ein wenn der Volumenstrom 0 l/s gesetzt wird.

v = isinf (u);

if v == 0
    
    y = u;

else 
    
    y = 0;
    
end

== matlab function closed circuit cooling tower/Leistungseinflüsse / influence on coolingpower/t_ia_ist /isnan ==
  data: u input inherited; y output inherited

function y = fcn(u)

%Verhindert die Fehlerausgabe bei Teilen durch den Wert 0 
%Dieser Zustand tritt ein wenn der Volumenstrom 0 l/s gesetzt wird.

v = isnan (u);

if v == 0
    
    y = u;

else 
    
    y = 0;
    
end

== matlab function closed circuit cooling tower/Verbrauch / consumption/Verdunstung/Verdunstungsmenge ==
  data: h_le input inherited; mdot input inherited; x_fl output inherited; qdot input inherited; t_ie input inherited; x_le input inherited; t_tau input inherited; p input inherited
function x_fl = fcn(h_le, mdot, qdot, t_ie, x_le, t_tau, p)

cp_lt = 1.006;
cp_d = 1.861;
cp_w = 4.19;
dhv0 = 2500;
tmax = t_ie;
tmin = t_tau;
t_zw = 15;
phi_luftaus = 100;
m = 1;


% Vorbedingung qdot muss positiv sein um eine Verdunstung zu gewährleisten ansonsten ist es ein Kondensation
if qdot < 0
    
    x_luftaus = 0;
    
else
    % Luftaustrittstemperaturberechnung, Halbierungsverfahren
        t_luftaus = (tmax+tmin)/2;
    
    % Absolute Feuchte-Berechnung Lufteintritt
        ps_luftaus = 611*exp((-1.91275)*10^(-4)+7.258*10^(-2)*t_luftaus-2.939*10^(-4)*t_luftaus^2+9.841*10^(-7)*t_luftaus^3-1.92*10^(-9)*t_luftaus^4);
        x_luftaus = (0.622*(phi_luftaus/100)*ps_luftaus)/(p-(phi_luftaus/100)*ps_luftaus);

    % Enthalpie Luftaustritt mit dem schon berechneten Qpkt
        h_la = qdot/mdot + (x_luftaus-x_le)*cp_w*t_zw + h_le;
    
    % Austrittstemperatur 
        tlab = (h_la - x_luftaus*dhv0)/(cp_lt + x_luftaus*cp_d);

    % Beginn der Schleife 
    % (t_luftaus - tlab) < 0,001 und > -0,001 ist die Austrittstemperatur gefunden
    %  t_luftaus < tlab  tmin = t_luftaus
    %  t_luftaus > tlab  tmax = t_luftaus
        while (t_luftaus - tlab)>0.001 || (t_luftaus - tlab) < -0.001 && m < 30
    
            if t_luftaus < tlab
        
                tmin = t_luftaus;
    
            else
        
                tmax = t_luftaus;
    
            end
    
            % Luftaustrittstemperaturberechnung, Halbierungsverfahren
                t_luftaus = (tmax+tmin)/2;
    
            % Absolute Feuchte-Berechnung Lufteintritt
                ps_luftaus = 611*exp((-1.91275)*10^(-4)+7.258*10^(-2)*t_luftaus-2.939*10^(-4)*t_luftaus^2+9.841*10^(-7)*t_luftaus^3-1.92*10^(-9)*t_luftaus^4);
                x_luftaus = (0.622*(phi_luftaus/100)*ps_luftaus)/(p-(phi_luftaus/100)*ps_luftaus);
        
            % Enthalpie Luftaustritt mit dem schon berechneten Qpkt
                h_la = qdot/mdot + (x_luftaus-x_le)*cp_w*t_zw + h_le;
        
            % Austrittstemperatur 
                tlab = (h_la - x_luftaus*dhv0)/(cp_lt + x_luftaus*cp_d);
        
            % Schleifenzähler
                m = m + 1;
    
        end

end

x_fl = x_luftaus-x_le;
